simulink model "One_3Ph_Induction_Motor"  (R2024a)
settings: Solver=ode23tb  StartTime=0.0  StopTime=10.0  MaxStep=1e-4  RelTol=1e-3
libraries: spsACVoltageSourceLib x9, spsAsynchronousMachineSIUnitsLib x3, spsGroundLib x3, sps_lib x1
settings Model: Creator=91889  LastModifiedBy=91889

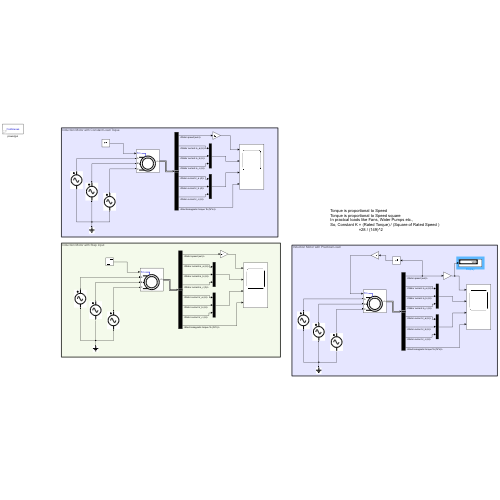
[thumbnail: Simulink's stored preview of the top-level diagram]
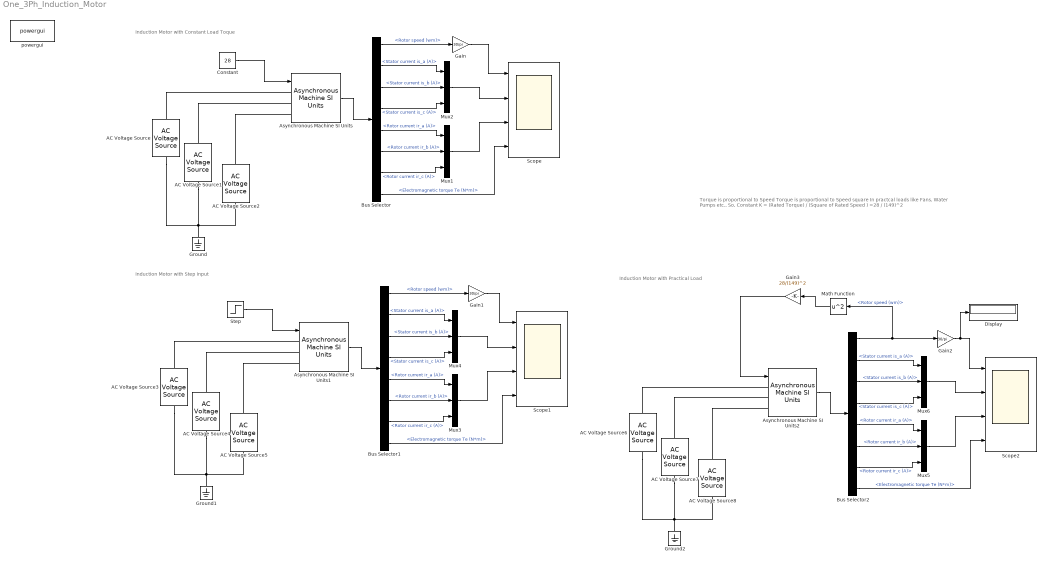
== system One_3Ph_Induction_Motor ==
  note: Torque is proportional to Speed
      | Torque is proportional to Speed square
      | In practcal loads like Fans, Water Pumps etc.,
      | So, Constant K = (Rated Torque) / (Square of Rated Speed )
      | =28 / (149)^2
  note: Induction Motor with Practical Load
  note: Induction Motor with Step input
  note: Induction Motor with Constant Load Toque
  AC Voltage Source : spsACVoltageSourceLib/AC Voltage Source  Amplitude=327  Phase=0  Frequency=50  SampleTime=0  Measurements=None  BusType=swing  Pref=10e3  Qref=0  Qmin=-inf  Qmax=+inf
  AC Voltage Source1 : spsACVoltageSourceLib/AC Voltage Source  Amplitude=327  Phase=-120  Frequency=50  SampleTime=0  Measurements=None  BusType=swing  Pref=10e3  Qref=0  Qmin=-inf  Qmax=+inf
  AC Voltage Source2 : spsACVoltageSourceLib/AC Voltage Source  Amplitude=327  Phase=120  Frequency=50  SampleTime=0  Measurements=None  BusType=swing  Pref=10e3  Qref=0  Qmin=-inf  Qmax=+inf
  AC Voltage Source3 : spsACVoltageSourceLib/AC Voltage Source  Amplitude=327  Phase=0  Frequency=50  SampleTime=0  Measurements=None  BusType=swing  Pref=10e3  Qref=0  Qmin=-inf  Qmax=+inf
  AC Voltage Source4 : spsACVoltageSourceLib/AC Voltage Source  Amplitude=327  Phase=-120  Frequency=50  SampleTime=0  Measurements=None  BusType=swing  Pref=10e3  Qref=0  Qmin=-inf  Qmax=+inf
  AC Voltage Source5 : spsACVoltageSourceLib/AC Voltage Source  Amplitude=327  Phase=120  Frequency=50  SampleTime=0  Measurements=None  BusType=swing  Pref=10e3  Qref=0  Qmin=-inf  Qmax=+inf
  AC Voltage Source6 : spsACVoltageSourceLib/AC Voltage Source  Amplitude=327  Phase=0  Frequency=50  SampleTime=0  Measurements=None  BusType=swing  Pref=10e3  Qref=0  Qmin=-inf  Qmax=+inf
  AC Voltage Source7 : spsACVoltageSourceLib/AC Voltage Source  Amplitude=327  Phase=-120  Frequency=50  SampleTime=0  Measurements=None  BusType=swing  Pref=10e3  Qref=0  Qmin=-inf  Qmax=+inf
  AC Voltage Source8 : spsACVoltageSourceLib/AC Voltage Source  Amplitude=327  Phase=120  Frequency=50  SampleTime=0  Measurements=None  BusType=swing  Pref=10e3  Qref=0  Qmin=-inf  Qmax=+inf
  Asynchronous Machine SI Units : spsAsynchronousMachineSIUnitsLib/Asynchronous Machine SI Units  RotorType=Squirrel-cage  PresetModel="15:  5.4 HP (4KW)   400 V  50Hz 1430 RPM"  MechanicalLoad=Torque Tm  ShowDetailedParameters=on  ReferenceFrame=Rotor  Units=SI  MeasurementBus=off  NominalParameters=[4000 400 50]  VoltageRatio=1  Stator=[1.405 0.005839]  Rotor=[1.395 0.005839]  Cage1=[0.4155 0.002066]  Cage2=[0.4168 0.0003495]  Lm=0.1722  Mechanical=[0.0131 0.002985 2]  PolePairs=2  InitialConditions=[0 0 0 0 0 0 0 0]  SimulateSaturation=off  Saturation=[14.03593122, 27.81365428, 53.79336849, 72.68890987, 97.98006896, 148.6815601, 215.7428561, 302.9841135, 428.7778367 ; 230, 322, 414, 460, 506, 552, 598, 644, 690]  LoadFlowParameters=1492000  TsPowergui=0  TsBlock=-1  IterativeModel=Trapezoidal non iterative  IterativeDiscreteModel=Trapezoidal non iterative  Pmec=1.492e+006
  Asynchronous Machine SI Units1 : spsAsynchronousMachineSIUnitsLib/Asynchronous Machine SI Units  RotorType=Squirrel-cage  PresetModel="15:  5.4 HP (4KW)   400 V  50Hz 1430 RPM"  MechanicalLoad=Torque Tm  ShowDetailedParameters=on  ReferenceFrame=Rotor  Units=SI  MeasurementBus=off  NominalParameters=[4000 400 50]  VoltageRatio=1  Stator=[1.405 0.005839]  Rotor=[1.395 0.005839]  Cage1=[0.4155 0.002066]  Cage2=[0.4168 0.0003495]  Lm=0.1722  Mechanical=[0.0131 0.002985 2]  PolePairs=2  InitialConditions=[0 0 0 0 0 0 0 0]  SimulateSaturation=off  Saturation=[14.03593122, 27.81365428, 53.79336849, 72.68890987, 97.98006896, 148.6815601, 215.7428561, 302.9841135, 428.7778367 ; 230, 322, 414, 460, 506, 552, 598, 644, 690]  LoadFlowParameters=1492000  TsPowergui=0  TsBlock=-1  IterativeModel=Trapezoidal non iterative  IterativeDiscreteModel=Trapezoidal non iterative  Pmec=1.492e+006
  Asynchronous Machine SI Units2 : spsAsynchronousMachineSIUnitsLib/Asynchronous Machine SI Units  RotorType=Squirrel-cage  PresetModel="15:  5.4 HP (4KW)   400 V  50Hz 1430 RPM"  MechanicalLoad=Torque Tm  ShowDetailedParameters=on  ReferenceFrame=Rotor  Units=SI  MeasurementBus=off  NominalParameters=[4000 400 50]  VoltageRatio=1  Stator=[1.405 0.005839]  Rotor=[1.395 0.005839]  Cage1=[0.4155 0.002066]  Cage2=[0.4168 0.0003495]  Lm=0.1722  Mechanical=[0.0131 0.002985 2]  PolePairs=2  InitialConditions=[0 0 0 0 0 0 0 0]  SimulateSaturation=off  Saturation=[14.03593122, 27.81365428, 53.79336849, 72.68890987, 97.98006896, 148.6815601, 215.7428561, 302.9841135, 428.7778367 ; 230, 322, 414, 460, 506, 552, 598, 644, 690]  LoadFlowParameters=1492000  TsPowergui=0  TsBlock=-1  IterativeModel=Trapezoidal non iterative  IterativeDiscreteModel=Trapezoidal non iterative  Pmec=1.492e+006
  Bus Selector : BusSelector  OutputSignals=Mechanical.Rotor speed (wm),Stator measurements.Stator current is_a (A),Stator measurements.Stator current is_b (A),Stator measurements.Stator current is_c (A),Rotor measurements.Rotor current ir_a (A),Rotor measurements.Rotor current ir_b (A),Rotor measurements.Rotor current ir_c (A),Mechanical.Electromagnetic torque Te (N*m)
  Bus Selector1 : BusSelector  OutputSignals=Mechanical.Rotor speed (wm),Stator measurements.Stator current is_a (A),Stator measurements.Stator current is_b (A),Stator measurements.Stator current is_c (A),Rotor measurements.Rotor current ir_a (A),Rotor measurements.Rotor current ir_b (A),Rotor measurements.Rotor current ir_c (A),Mechanical.Electromagnetic torque Te (N*m)
  Bus Selector2 : BusSelector  OutputSignals=Mechanical.Rotor speed (wm),Stator measurements.Stator current is_a (A),Stator measurements.Stator current is_b (A),Stator measurements.Stator current is_c (A),Rotor measurements.Rotor current ir_a (A),Rotor measurements.Rotor current ir_b (A),Rotor measurements.Rotor current ir_c (A),Mechanical.Electromagnetic torque Te (N*m)
  Constant : Constant  Value=28
  Display : Display
  Gain : Gain  Gain=30/pi
  Gain1 : Gain  Gain=30/pi
  Gain2 : Gain  Gain=30/pi
  Gain3 : Gain  Gain=28/(149)^2
  Ground : spsGroundLib/Ground  LConnTagsString=a
  Ground1 : spsGroundLib/Ground  LConnTagsString=a
  Ground2 : spsGroundLib/Ground  LConnTagsString=a
  Math Function : Math  Operator=square
  Mux{1..6} (6 alike) : Mux  Inputs=3
  Scope : Scope  NumInputPorts=4
  Scope1 : Scope  NumInputPorts=4
  Scope2 : Scope  NumInputPorts=4
  Step : Step  Time=5  After=28  SampleTime=0
  powergui : sps_lib/powergui  Priority=1  SimulationMode=Continuous  SampleTime=50e-6  frequency=60  Iterations=50  frequencyindice=50  Pbase=100e6  ErrMax=1e-4  UnitsV=kV  UnitsW=MW  buscounter=0  FunctionMessages=off  echomessages=off  EnableUseOfTLC=off  CurrentSourceSwitches=off  DisableSnubberDevices=off  DisableRonSwitches=off  DisableVfSwitches=off  DisplayEquations=off  AutomaticDiscreteSolvers=off  SolverType=Tustin/Backward Euler (TBE)  Interpol=off  ExternalGateDelay=off  methode=off  Ts=100  x0status=blocks  SPID=on  SwTol=0  HookPort=off  NonlinearTolerance=1e-4  nMaxIteration=100  ContinueOnMaxIteration=off  RestoreLinks=warning  ResistiveCurrentMeasurement=off  Frange=[0:2:500]  Ylog=off  Xlog=on  ShowGrid=off  save=off  variable=ZData  structure=0  ZoomFFT=off  StartTime=0.0  cycles=1  DisplayStyle=1  fundamental=60  FreqAxis=off  MaxFrequency=1000  frequencyindicesteady=1  RmsSteady=1  display=off
  wires:
  Asynchronous Machine SI Units/1 -> Bus Selector/1
  Bus Selector/2 -> Mux2/1  "<Stator current is_a (A)>"
  Bus Selector/3 -> Mux2/2  "<Stator current is_b (A)>"
  Bus Selector/4 -> Mux2/3  "<Stator current is_c (A)>"
  Bus Selector/5 -> Mux1/1  "<Rotor current ir_a (A)>"
  Bus Selector/6 -> Mux1/2  "<Rotor current ir_b (A)>"
  Bus Selector/7 -> Mux1/3  "<Rotor current ir_c (A)>"
  Mux2/1 -> Scope/2
  Mux1/1 -> Scope/3
  Bus Selector/8 -> Scope/4  "<Electromagnetic torque Te (N*m)>"
  Constant/1 -> Asynchronous Machine SI Units/1
  Step/1 -> Asynchronous Machine SI Units1/1
  Bus Selector1/8 -> Scope1/4  "<Electromagnetic torque Te (N*m)>"
  Mux4/1 -> Scope1/2
  Bus Selector1/2 -> Mux4/1  "<Stator current is_a (A)>"
  Bus Selector1/6 -> Mux3/2  "<Rotor current ir_b (A)>"
  Mux3/1 -> Scope1/3
  Bus Selector1/5 -> Mux3/1  "<Rotor current ir_a (A)>"
  Bus Selector1/3 -> Mux4/2  "<Stator current is_b (A)>"
  Asynchronous Machine SI Units1/1 -> Bus Selector1/1
  Bus Selector1/4 -> Mux4/3  "<Stator current is_c (A)>"
  Bus Selector1/7 -> Mux3/3  "<Rotor current ir_c (A)>"
  Bus Selector2/7 -> Mux5/3  "<Rotor current ir_c (A)>"
  Mux5/1 -> Scope2/3
  Bus Selector2/5 -> Mux5/1  "<Rotor current ir_a (A)>"
  Bus Selector2/3 -> Mux6/2  "<Stator current is_b (A)>"
  Bus Selector2/8 -> Scope2/4  "<Electromagnetic torque Te (N*m)>"
  Bus Selector2/6 -> Mux5/2  "<Rotor current ir_b (A)>"
  Mux6/1 -> Scope2/2
  Asynchronous Machine SI Units2/1 -> Bus Selector2/1
  Bus Selector2/2 -> Mux6/1  "<Stator current is_a (A)>"
  Gain3/1 -> Asynchronous Machine SI Units2/1
  Bus Selector2/4 -> Mux6/3  "<Stator current is_c (A)>"
  Bus Selector/1 -> Gain/1  "<Rotor speed (wm)>"
  Gain/1 -> Scope/1
  Bus Selector1/1 -> Gain1/1  "<Rotor speed (wm)>"
  Gain1/1 -> Scope1/1
  Bus Selector2/1 -> Math Function/1, Gain2/1  "<Rotor speed (wm)>"
  Gain2/1 -> Display/1, Scope2/1
  Math Function/1 -> Gain3/1
  connections:
  AC Voltage Source/RConn1 -- Asynchronous Machine SI Units/LConn1
  AC Voltage Source1/RConn1 -- Asynchronous Machine SI Units/LConn2
  AC Voltage Source2/RConn1 -- Asynchronous Machine SI Units/LConn3
  AC Voltage Source/LConn1 -- AC Voltage Source1/LConn1 -- Ground/LConn1 -- AC Voltage Source2/LConn1
  AC Voltage Source3/LConn1 -- AC Voltage Source4/LConn1 -- Ground1/LConn1 -- AC Voltage Source5/LConn1
  AC Voltage Source4/RConn1 -- Asynchronous Machine SI Units1/LConn2
  AC Voltage Source3/RConn1 -- Asynchronous Machine SI Units1/LConn1
  AC Voltage Source5/RConn1 -- Asynchronous Machine SI Units1/LConn3
  AC Voltage Source8/LConn1 -- AC Voltage Source7/LConn1 -- Ground2/LConn1 -- AC Voltage Source6/LConn1
  AC Voltage Source8/RConn1 -- Asynchronous Machine SI Units2/LConn3
  AC Voltage Source7/RConn1 -- Asynchronous Machine SI Units2/LConn2
  AC Voltage Source6/RConn1 -- Asynchronous Machine SI Units2/LConn1
